simulink model "motor_model"  (R2017a)
settings: Solver=ode45  StartTime=0.0  StopTime=3  RelTol=1e-3  EnableMultiTasking=on
values from neighbouring files (symbols this model uses):
  motor = gm9434    [motor_code.m]
undefined symbols (not defined in the file or in its folder): current_ctrl, joint, position_ctrl, speed_ctrl, vest
libraries: simulink x6
settings Model: Creator=rodrigo  LastModifiedBy=rodrigo
settings DataIOCC: LimitDataPoints=on  SaveFormat=Array
settings OptimizationCC: LifeSpan=inf
settings DebuggingCC: UnderspecifiedInitializationDetection=Classic  MergeDetectMultiDrivingBlocksExec=none  StateNameClashWarn=warning  SFUnexpectedBacktrackingDiag=warning  SFNoUnconditionalDefaultTransitionDiag=warning  SFExecutionAtInitializationDiag=none
settings HardwareCC: ProdBitPerPointer=32  ProdBitPerSizeT=32  ProdBitPerPtrDiffT=32  ProdLargestAtomicFloat=None  ProdIntDivRoundTo=Undefined  ProdEndianess=Unspecified  ProdWordSize=32  ProdHWDeviceType=32-bit Generic
settings ModelReferenceCC: PropagateSignalLabelsOutOfModel=off
settings GRTTargetCC: TargetLangStandard=C89/C90 (ANSI)  GeneratePreprocessorConditionals=Disable all
settings ConfigComp: CovMetricSettings=dw  CovHtmlReporting=on  CovSaveCumulativeToWorkspaceVar=on  CovSaveSingleToWorkspaceVar=on  CovExternalEMLEnable=off

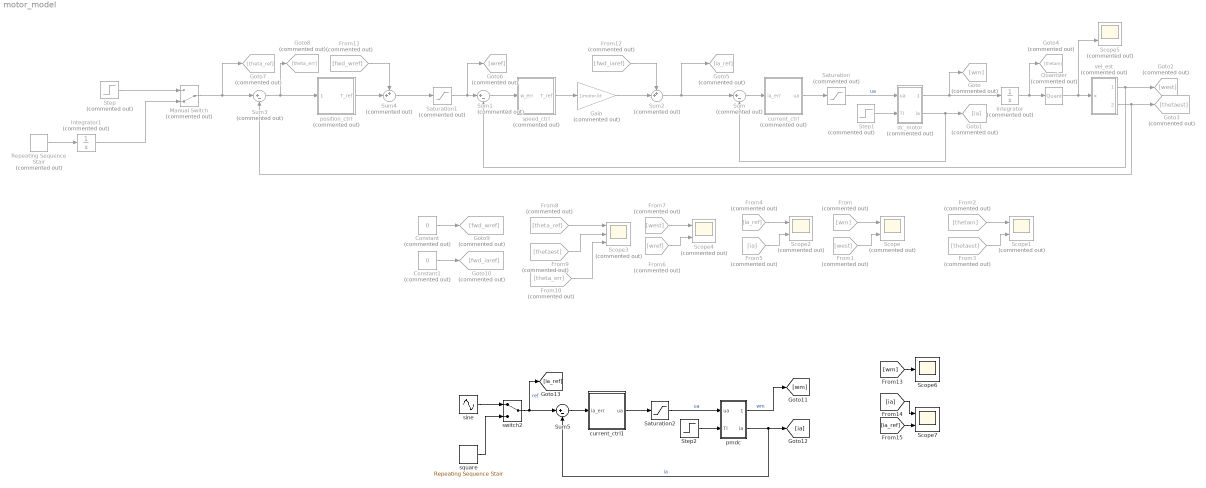
== system motor_model ==
  Constant : Constant  Commented=on  Value=0
  Constant1 : Constant  Commented=on  Value=0
  From : From  Commented=on  GotoTag=wm
  From1 : From  Commented=on  GotoTag=west
  From10 : From  Commented=on  GotoTag=theta_err
  From11 : From  Commented=on  GotoTag=fwd_wref
  From12 : From  Commented=on  GotoTag=fwd_iaref
  From2 : From  Commented=on  GotoTag=thetam
  From3 : From  Commented=on  GotoTag=thetaest
  From4 : From  Commented=on  GotoTag=ia_ref
  From5 : From  Commented=on  GotoTag=ia
  From6 : From  Commented=on  GotoTag=wref
  From7 : From  Commented=on  GotoTag=west
  From8 : From  Commented=on  GotoTag=theta_ref
  From9 : From  Commented=on  GotoTag=thetaest
  Gain : Gain  Commented=on  Gain=1/motor.kt
  Goto : Goto  Commented=on  GotoTag=wm
  Goto1 : Goto  Commented=on  GotoTag=ia
  Goto10 : Goto  Commented=on  GotoTag=fwd_iaref
  Goto2 : Goto  Commented=on  GotoTag=west
  Goto3 : Goto  Commented=on  GotoTag=thetaest
  Goto4 : Goto  Commented=on  GotoTag=thetam
  Goto5 : Goto  Commented=on  GotoTag=ia_ref
  Goto6 : Goto  Commented=on  GotoTag=wref
  Goto7 : Goto  Commented=on  GotoTag=theta_ref
  Goto8 : Goto  Commented=on  GotoTag=theta_err
  Goto9 : Goto  Commented=on  GotoTag=fwd_wref
  Integrator : Integrator  Commented=on
  Integrator1 : Integrator  Commented=on
  Manual Switch : ManualSwitch  Commented=on  CurrentSetting=0
  Quantizer : Quantizer  Commented=on  QuantizationInterval=encoder
  Repeating Sequence Stair : simulink/Sources/Repeating Sequence Stair  Commented=on  OutValues=[0,100,100,100,100,0,0, -100,-100,-100,-100,-100,-100,-100,-100,0,0,100,100,100,100]  tsamp=1  OutMin=[]  OutMax=[]  OutDataTypeStr=double  OutputDataTypeScalingMode=double  OutDataType=fixdt(0,8)  ConRadixGroup=Best Precision: Vector-wise  OutScaling=2^-12
  Saturation : Saturate  Commented=on  UpperLimit=12  LowerLimit=-12
  Saturation1 : Saturate  Commented=on  UpperLimit=motor.max_speed  LowerLimit=-motor.max_speed
  Saturation2 : Saturate  UpperLimit=12  LowerLimit=-12
  Scope{,1..2,4..5} (5 alike) : Scope  Commented=on  NumInputPorts=2
  Scope3 : Scope  Commented=on  NumInputPorts=3
  Scope6 : Scope
  Scope7 : Scope  NumInputPorts=2
  Step : Step  Commented=on  After=800  SampleTime=0
  Step1 : Step  Commented=on  After=0  SampleTime=0  ZeroCross=off
  Step2 : Step  After=0  SampleTime=0  ZeroCross=off
  Sum : Sum  Commented=on  Inputs=|+-
  Sum1 : Sum  Commented=on  Inputs=|+-
  Sum2 : Sum  Commented=on  Inputs=++|
  Sum3 : Sum  Commented=on  Inputs=|+-
  Sum4 : Sum  Commented=on  Inputs=++|
  Sum5 : Sum  Inputs=|+-
  current_ctrl : Subsystem  Commented=on
  current_ctrl1 : Subsystem
  dc_motor : Subsystem  Commented=on
  pmdc : Subsystem
  position_ctrl : Subsystem  Commented=on
  sine : Sin  Frequency=50*2*pi  SampleTime=0
  speed_ctrl : Subsystem  Commented=on
  square : simulink/Sources/Repeating Sequence Stair  OutValues=[1 -1 1 -1]  tsamp=1  OutMin=[]  OutMax=[]  OutDataTypeStr=double  OutputDataTypeScalingMode=double  OutDataType=fixdt(0,8)  ConRadixGroup=Best Precision: Vector-wise  OutScaling=2^-12
  switch2 : ManualSwitch
  vel_est : Subsystem  Commented=on
  wires:
  From/1 -> Scope/1
  From1/1 -> Scope/2
  dc_motor/2(ia) -> Goto1/1, Sum/2
  Step1/1 -> dc_motor/2(Tl)
  Saturation/1 -> dc_motor/1(ua)  "ua"
  dc_motor/1(wm) -> Integrator/1, Goto/1
  Integrator/1 -> Quantizer/1, Goto4/1
  Quantizer/1 -> Scope5/2, vel_est/1(x)
  From2/1 -> Scope1/1
  From3/1 -> Scope1/2
  vel_est/2(xest) -> Sum3/2, Goto3/1
  From4/1 -> Scope2/1
  From5/1 -> Scope2/2
  Sum/1 -> current_ctrl/1(ia_err)
  current_ctrl/1(ua) -> Saturation/1
  speed_ctrl/1(T_ref) -> Gain/1
  Sum1/1 -> speed_ctrl/1(w_err)
  From7/1 -> Scope4/1
  From6/1 -> Scope4/2
  Sum2/1 -> Goto5/1, Sum/1
  Gain/1 -> Sum2/2
  From12/1 -> Sum2/1
  Sum3/1 -> Goto8/1, position_ctrl/1(theta_err)
  From8/1 -> Scope3/1
  From10/1 -> Scope3/3
  vel_est/1(vest) -> Sum1/2, Goto2/1
  From9/1 -> Scope3/2
  Saturation1/1 -> Goto6/1, Sum1/1
  From11/1 -> Sum4/1
  position_ctrl/1(T_ref) -> Sum4/2
  Sum4/1 -> Saturation1/1
  Constant/1 -> Goto9/1
  Constant1/1 -> Goto10/1
  Repeating Sequence Stair/1 -> Integrator1/1
  Manual Switch/1 -> Goto7/1, Sum3/1
  Step/1 -> Manual Switch/1
  Integrator1/1 -> Manual Switch/2
  pmdc/2(ia) -> [ia], Sum5/2  "ia"
  Step2/1 -> pmdc/2(Tl)
  current_ctrl1/1(ua) -> Saturation2/1
  Sum5/1 -> current_ctrl1/1(ia_err)
  pmdc/1(wm) -> [wm]  "wm"
  Saturation2/1 -> pmdc/1(ua)  "ua"
  [wm] -> Scope6/1
  [ia] -> Scope7/1
  [ia_ref] -> Scope7/2
  sine/1 -> switch2/1
  square/1 -> switch2/2
  switch2/1 -> [ia_ref], Sum5/1  "ref"

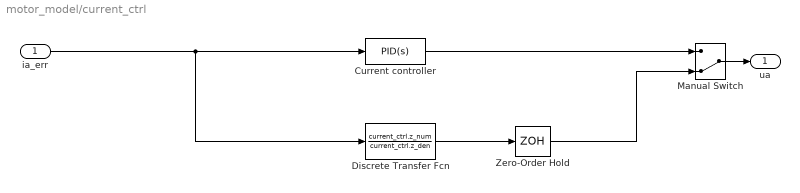
== system motor_model/current_ctrl ==
  ia_err : Inport
  Current controller : simulink/Continuous/PID Controller  Controller=PID  TimeDomain=Continuous-time  SampleTime=-1  IntegratorMethod=Forward Euler  FilterMethod=Forward Euler  Form=Parallel  UseFilter=off  ControllerParametersSource=internal  P=current_ctrl.kp  I=current_ctrl.ki  D=0  N=100  InitialConditionSource=internal  InitialConditionForIntegrator=0  InitialConditionForFilter=0  ExternalReset=none  ZeroCross=off  LimitOutput=on  UpperSaturationLimit=12  LowerSaturationLimit=-12  LinearizeAsGain=off  AntiWindupMode=back-calculation  Kb=1  TrackingMode=off  Kt=1  PParamMin=[]  PParamMax=[]  IParamMin=[]  IParamMax=[]  DParamMin=[]  DParamMax=[]  NParamMin=[]  NParamMax=[]  KbParamMin=[]  KbParamMax=[]  KtParamMin=[]  KtParamMax=[]  POutMin=[]  POutMax=[]  IOutMin=[]  IOutMax=[]  DOutMin=[]  DOutMax=[]  NOutMin=[]  NOutMax=[]  KbOutMin=[]  KbOutMax=[]  KtOutMin=[]  KtOutMax=[]  IntegratorOutMin=[]  IntegratorOutMax=[]  FilterOutMin=[]  FilterOutMax=[]  SumOutMin=[]  SumOutMax=[]  SumI1OutMin=[]  SumI1OutMax=[]  SumI2OutMin=[]  SumI2OutMax=[]  SumI3OutMin=[]  SumI3OutMax=[]  SumDOutMin=[]  SumDOutMax=[]  SaturationOutMin=[]  SaturationOutMax=[]  IntegratorContinuousStateAttributes=''  IntegratorStateMustResolveToSignalObject=off  IntegratorRTWStateStorageClass=Auto  FilterContinuousStateAttributes=''  FilterStateMustResolveToSignalObject=off  FilterRTWStateStorageClass=Auto  DifferentiatorICPrevScaledInput=0  DifferentiatorOutMin=[]  DifferentiatorOutMax=[]  InitialConditionSetting=State (most efficient)
  Discrete Transfer Fcn : DiscreteTransferFcn  Numerator=current_ctrl.z_num  Denominator=current_ctrl.z_den  SampleTime=current_ctrl.Ts
  Manual Switch : ManualSwitch  CurrentSetting=0
  Zero-Order Hold : ZeroOrderHold  SampleTime=-1
  ua : Outport
  wires:
  ia_err/1 -> Discrete Transfer Fcn/1, Current controller/1
  Current controller/1 -> Manual Switch/1
  Discrete Transfer Fcn/1 -> Zero-Order Hold/1
  Zero-Order Hold/1 -> Manual Switch/2
  Manual Switch/1 -> ua/1

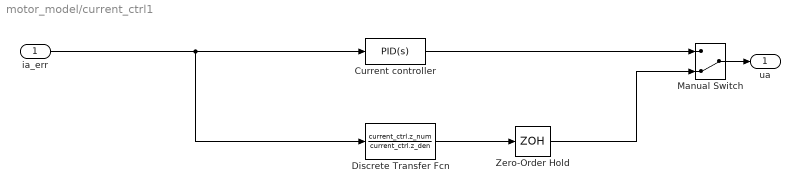
== system motor_model/current_ctrl1 ==
  ia_err : Inport
  Current controller : simulink/Continuous/PID Controller  Controller=PID  TimeDomain=Continuous-time  SampleTime=-1  IntegratorMethod=Forward Euler  FilterMethod=Forward Euler  Form=Parallel  UseFilter=off  ControllerParametersSource=internal  P=current_ctrl.kp  I=current_ctrl.ki  D=0  N=100  InitialConditionSource=internal  InitialConditionForIntegrator=0  InitialConditionForFilter=0  ExternalReset=none  ZeroCross=off  LimitOutput=on  UpperSaturationLimit=12  LowerSaturationLimit=-12  LinearizeAsGain=off  AntiWindupMode=back-calculation  Kb=1  TrackingMode=off  Kt=1  PParamMin=[]  PParamMax=[]  IParamMin=[]  IParamMax=[]  DParamMin=[]  DParamMax=[]  NParamMin=[]  NParamMax=[]  KbParamMin=[]  KbParamMax=[]  KtParamMin=[]  KtParamMax=[]  POutMin=[]  POutMax=[]  IOutMin=[]  IOutMax=[]  DOutMin=[]  DOutMax=[]  NOutMin=[]  NOutMax=[]  KbOutMin=[]  KbOutMax=[]  KtOutMin=[]  KtOutMax=[]  IntegratorOutMin=[]  IntegratorOutMax=[]  FilterOutMin=[]  FilterOutMax=[]  SumOutMin=[]  SumOutMax=[]  SumI1OutMin=[]  SumI1OutMax=[]  SumI2OutMin=[]  SumI2OutMax=[]  SumI3OutMin=[]  SumI3OutMax=[]  SumDOutMin=[]  SumDOutMax=[]  SaturationOutMin=[]  SaturationOutMax=[]  IntegratorContinuousStateAttributes=''  IntegratorStateMustResolveToSignalObject=off  IntegratorRTWStateStorageClass=Auto  FilterContinuousStateAttributes=''  FilterStateMustResolveToSignalObject=off  FilterRTWStateStorageClass=Auto  DifferentiatorICPrevScaledInput=0  DifferentiatorOutMin=[]  DifferentiatorOutMax=[]  InitialConditionSetting=State (most efficient)
  Discrete Transfer Fcn : DiscreteTransferFcn  Numerator=current_ctrl.z_num  Denominator=current_ctrl.z_den  SampleTime=current_ctrl.Ts
  Manual Switch : ManualSwitch  CurrentSetting=0
  Zero-Order Hold : ZeroOrderHold  SampleTime=-1
  ua : Outport
  wires:
  ia_err/1 -> Discrete Transfer Fcn/1, Current controller/1
  Current controller/1 -> Manual Switch/1
  Discrete Transfer Fcn/1 -> Zero-Order Hold/1
  Zero-Order Hold/1 -> Manual Switch/2
  Manual Switch/1 -> ua/1

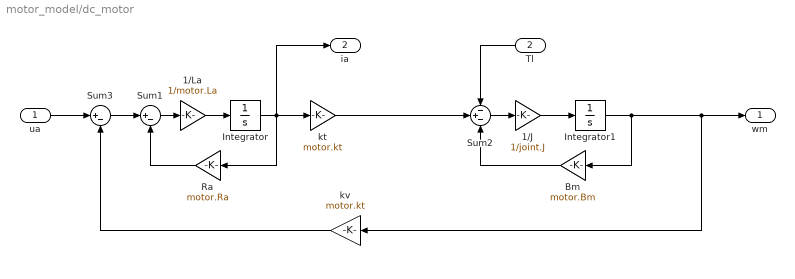
== system motor_model/dc_motor ==
  ua : Inport
  Tl : Inport  Port=2
  1/J : Gain  Gain=1/joint.J
  1/La : Gain  Gain=1/motor.La
  Bm : Gain  Gain=motor.Bm
  Integrator : Integrator  ZeroCross=off
  Integrator1 : Integrator
  Ra : Gain  Gain=motor.Ra
  Sum1 : Sum  Inputs=|+-
  Sum2 : Sum  Inputs=-+-
  Sum3 : Sum  Inputs=|+-
  kt : Gain  Gain=motor.kt
  kv : Gain  Gain=motor.kt
  wm : Outport
  ia : Outport  Port=2
  wires:
  1/J/1 -> Integrator1/1
  Sum2/1 -> 1/J/1
  Integrator1/1 -> Bm/1, wm/1, kv/1
  ua/1 -> Sum3/1
  Integrator/1 -> kt/1, Ra/1, ia/1
  Ra/1 -> Sum1/2
  1/La/1 -> Integrator/1
  Tl/1 -> Sum2/1
  kv/1 -> Sum3/2
  Sum3/1 -> Sum1/1
  Sum1/1 -> 1/La/1
  kt/1 -> Sum2/2
  Bm/1 -> Sum2/3

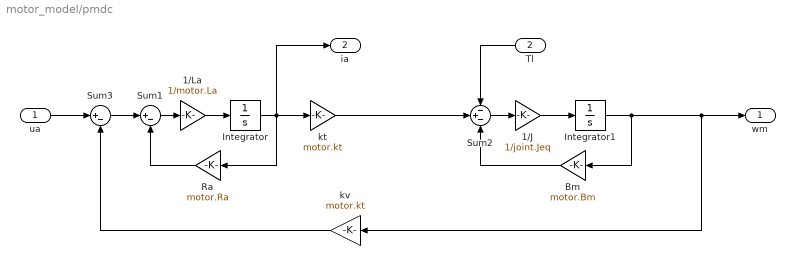
== system motor_model/pmdc ==
  ua : Inport
  Tl : Inport  Port=2
  1/J : Gain  Gain=1/joint.Jeq
  1/La : Gain  Gain=1/motor.La
  Bm : Gain  Gain=motor.Bm
  Integrator : Integrator  ZeroCross=off
  Integrator1 : Integrator
  Ra : Gain  Gain=motor.Ra
  Sum1 : Sum  Inputs=|+-
  Sum2 : Sum  Inputs=-+-
  Sum3 : Sum  Inputs=|+-
  kt : Gain  Gain=motor.kt
  kv : Gain  Gain=motor.kt
  wm : Outport
  ia : Outport  Port=2
  wires:
  1/J/1 -> Integrator1/1
  Sum2/1 -> 1/J/1
  Integrator1/1 -> Bm/1, wm/1, kv/1
  ua/1 -> Sum3/1
  Integrator/1 -> kt/1, Ra/1, ia/1
  Ra/1 -> Sum1/2
  1/La/1 -> Integrator/1
  Tl/1 -> Sum2/1
  kv/1 -> Sum3/2
  Sum3/1 -> Sum1/1
  Sum1/1 -> 1/La/1
  kt/1 -> Sum2/2
  Bm/1 -> Sum2/3

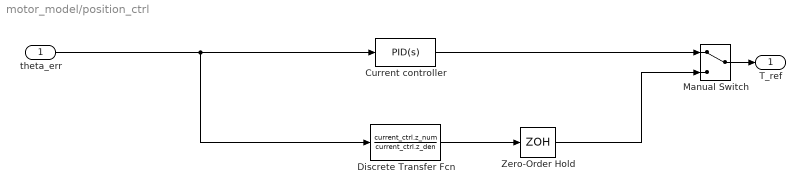
== system motor_model/position_ctrl ==
  theta_err : Inport
  Current controller : simulink/Continuous/PID Controller  Controller=PID  TimeDomain=Continuous-time  SampleTime=-1  IntegratorMethod=Forward Euler  FilterMethod=Forward Euler  Form=Ideal  UseFilter=off  ControllerParametersSource=internal  P=position_ctrl.kp*3  I=0.3  D=0  N=100  InitialConditionSource=internal  InitialConditionForIntegrator=0  InitialConditionForFilter=0  ExternalReset=none  ZeroCross=off  LimitOutput=on  UpperSaturationLimit=300  LowerSaturationLimit=-300  LinearizeAsGain=off  AntiWindupMode=back-calculation  Kb=1  TrackingMode=off  Kt=1  PParamMin=[]  PParamMax=[]  IParamMin=[]  IParamMax=[]  DParamMin=[]  DParamMax=[]  NParamMin=[]  NParamMax=[]  KbParamMin=[]  KbParamMax=[]  KtParamMin=[]  KtParamMax=[]  POutMin=[]  POutMax=[]  IOutMin=[]  IOutMax=[]  DOutMin=[]  DOutMax=[]  NOutMin=[]  NOutMax=[]  KbOutMin=[]  KbOutMax=[]  KtOutMin=[]  KtOutMax=[]  IntegratorOutMin=[]  IntegratorOutMax=[]  FilterOutMin=[]  FilterOutMax=[]  SumOutMin=[]  SumOutMax=[]  SumI1OutMin=[]  SumI1OutMax=[]  SumI2OutMin=[]  SumI2OutMax=[]  SumI3OutMin=[]  SumI3OutMax=[]  SumDOutMin=[]  SumDOutMax=[]  SaturationOutMin=[]  SaturationOutMax=[]  IntegratorContinuousStateAttributes=''  IntegratorStateMustResolveToSignalObject=off  IntegratorRTWStateStorageClass=Auto  FilterContinuousStateAttributes=''  FilterStateMustResolveToSignalObject=off  FilterRTWStateStorageClass=Auto  DifferentiatorICPrevScaledInput=0  DifferentiatorOutMin=[]  DifferentiatorOutMax=[]  InitialConditionSetting=State (most efficient)
  Discrete Transfer Fcn : DiscreteTransferFcn  Numerator=current_ctrl.z_num  Denominator=current_ctrl.z_den  SampleTime=current_ctrl.Ts
  Manual Switch : ManualSwitch
  Zero-Order Hold : ZeroOrderHold  SampleTime=-1
  T_ref : Outport
  wires:
  theta_err/1 -> Current controller/1, Discrete Transfer Fcn/1
  Current controller/1 -> Manual Switch/1
  Discrete Transfer Fcn/1 -> Zero-Order Hold/1
  Zero-Order Hold/1 -> Manual Switch/2
  Manual Switch/1 -> T_ref/1

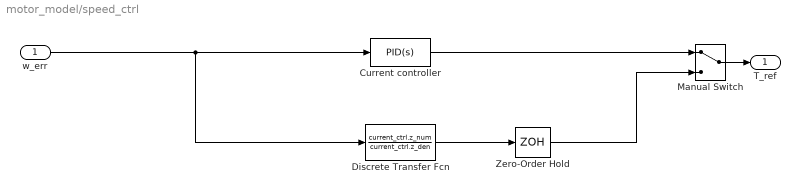
== system motor_model/speed_ctrl ==
  w_err : Inport
  Current controller : simulink/Continuous/PID Controller  Controller=PID  TimeDomain=Continuous-time  SampleTime=-1  IntegratorMethod=Forward Euler  FilterMethod=Forward Euler  Form=Ideal  UseFilter=off  ControllerParametersSource=internal  P=speed_ctrl.kp  I=speed_ctrl.ki  D=0  N=100  InitialConditionSource=internal  InitialConditionForIntegrator=0  InitialConditionForFilter=0  ExternalReset=none  ZeroCross=off  LimitOutput=on  UpperSaturationLimit=3  LowerSaturationLimit=-3  LinearizeAsGain=off  AntiWindupMode=back-calculation  Kb=1  TrackingMode=off  Kt=1  PParamMin=[]  PParamMax=[]  IParamMin=[]  IParamMax=[]  DParamMin=[]  DParamMax=[]  NParamMin=[]  NParamMax=[]  KbParamMin=[]  KbParamMax=[]  KtParamMin=[]  KtParamMax=[]  POutMin=[]  POutMax=[]  IOutMin=[]  IOutMax=[]  DOutMin=[]  DOutMax=[]  NOutMin=[]  NOutMax=[]  KbOutMin=[]  KbOutMax=[]  KtOutMin=[]  KtOutMax=[]  IntegratorOutMin=[]  IntegratorOutMax=[]  FilterOutMin=[]  FilterOutMax=[]  SumOutMin=[]  SumOutMax=[]  SumI1OutMin=[]  SumI1OutMax=[]  SumI2OutMin=[]  SumI2OutMax=[]  SumI3OutMin=[]  SumI3OutMax=[]  SumDOutMin=[]  SumDOutMax=[]  SaturationOutMin=[]  SaturationOutMax=[]  IntegratorContinuousStateAttributes=''  IntegratorStateMustResolveToSignalObject=off  IntegratorRTWStateStorageClass=Auto  FilterContinuousStateAttributes=''  FilterStateMustResolveToSignalObject=off  FilterRTWStateStorageClass=Auto  DifferentiatorICPrevScaledInput=0  DifferentiatorOutMin=[]  DifferentiatorOutMax=[]  InitialConditionSetting=State (most efficient)
  Discrete Transfer Fcn : DiscreteTransferFcn  Numerator=current_ctrl.z_num  Denominator=current_ctrl.z_den  SampleTime=current_ctrl.Ts
  Manual Switch : ManualSwitch
  Zero-Order Hold : ZeroOrderHold  SampleTime=-1
  T_ref : Outport
  wires:
  w_err/1 -> Current controller/1, Discrete Transfer Fcn/1
  Current controller/1 -> Manual Switch/1
  Discrete Transfer Fcn/1 -> Zero-Order Hold/1
  Zero-Order Hold/1 -> Manual Switch/2
  Manual Switch/1 -> T_ref/1

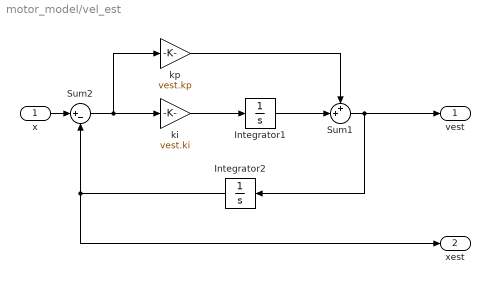
== system motor_model/vel_est ==
  x : Inport
  Integrator1 : Integrator
  Integrator2 : Integrator
  Sum1 : Sum  Inputs=++|
  Sum2 : Sum  Inputs=|+-
  ki : Gain  Gain=vest.ki
  kp : Gain  Gain=vest.kp
  vest : Outport
  xest : Outport  Port=2
  wires:
  ki/1 -> Integrator1/1
  Sum2/1 -> kp/1, ki/1
  Integrator2/1 -> xest/1, Sum2/2
  kp/1 -> Sum1/1
  Integrator1/1 -> Sum1/2
  x/1 -> Sum2/1
  Sum1/1 -> vest/1, Integrator2/1
